simulink model "model5_2_d"  (R2024b)
settings: Solver=VariableStepAuto  StartTime=0.0  StopTime=0.015  RelTol=1e-3
values from neighbouring files (symbols this model uses):
  Rd = [1, RS(1) - 1, -RS(1)]    [domaci5_3_d.m]
  Sd = RS(2:end)'    [domaci5_3_d.m]
  Ts = 0.001    [domaci5_3_d.m]
  Tsd = 1 / dcgain(minreal(1/Rsd * feedback(Gpd, Ssd/Rsd)))    [domaci5_3_d.m]
settings Model: Creator=neso  LastModifiedBy=neso

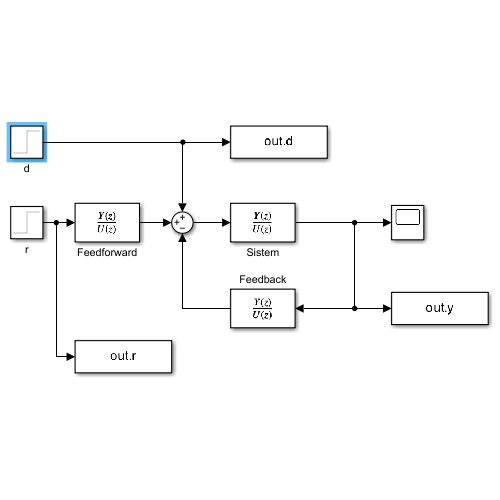
[thumbnail: Simulink's stored preview of the top-level diagram]
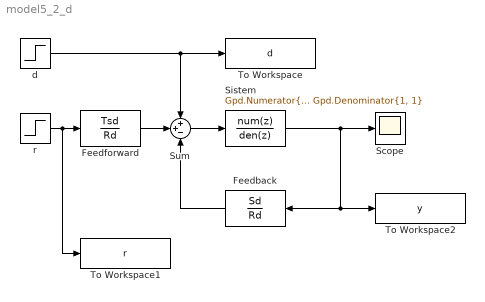
== system model5_2_d ==
  Feedback : DiscreteTransferFcn  Numerator=Sd  Denominator=Rd
  Feedforward : DiscreteTransferFcn  Numerator=Tsd  Denominator=Rd
  Scope : Scope
  Sistem : DiscreteTransferFcn  Numerator=Gpd.Numerator{1, 1}  Denominator=Gpd.Denominator{1, 1}
  Sum : Sum  Inputs=++-
  To Workspace : ToWorkspace  VariableName=d  SaveFormat=Timeseries  SampleTime=-1
  To Workspace1 : ToWorkspace  VariableName=r  SaveFormat=Timeseries  SampleTime=-1
  To Workspace2 : ToWorkspace  VariableName=y  SaveFormat=Timeseries  SampleTime=-1
  d : Step  Time=0.007  SampleTime=Ts
  r : Step  Time=0  After=5  SampleTime=Ts
  wires:
  Sum/1 -> Sistem/1
  r/1 -> To Workspace1/1, Feedforward/1
  Sistem/1 -> To Workspace2/1, Feedback/1, Scope/1
  Feedforward/1 -> Sum/2
  Feedback/1 -> Sum/3
  d/1 -> To Workspace/1, Sum/1
